simulink model "fly_gaze_sim"  (R2022a)
settings: Solver=ode45  StartTime=0.0  StopTime=t_run  MaxStep=1e-4  RelTol=1e-6
values from neighbouring files (symbols this model uses):
  frequency = test_frequencies(i)    [generate_data.m]
  t_run = 1 + 10/frequency    [generate_data.m]
libraries: simulink x1
settings Model: Creator=Ben  LastModifiedBy=Ben

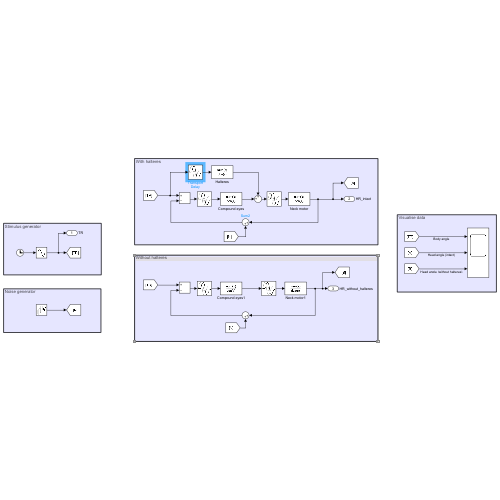
[thumbnail: Simulink's stored preview of the top-level diagram]
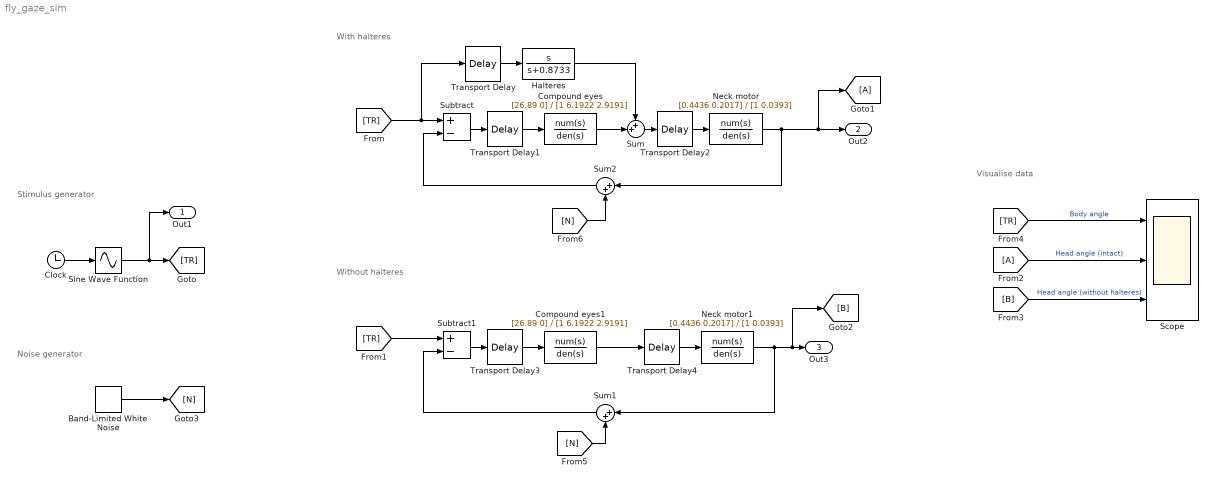
== system fly_gaze_sim ==
  note: Noise generator
  note: Visualise data
  note: With halteres
  note: Stimulus generator
  note: Without halteres
  Band-Limited White Noise : simulink/Sources/Band-Limited White Noise  Cov=[1/t_run]  Ts=0.000001*t_run  seed=[23341]
  Clock : Clock
      settings: Decimation=1000
  Compound eyes : TransferFcn  Numerator=[26.89 0]  Denominator=[1 6.1922 2.9191]
  Compound eyes1 : TransferFcn  Numerator=[26.89 0]  Denominator=[1 6.1922 2.9191]
  From2 : From
  Goto1 : Goto
  Halteres : TransferFcn  Numerator=[1 0]  Denominator=[1 0.8733]
  Neck motor : TransferFcn  Numerator=[0.4436 0.2017]  Denominator=[1 0.0393]
  Neck motor1 : TransferFcn  Numerator=[0.4436 0.2017]  Denominator=[1 0.0393]
  Scope : Scope  NumInputPorts=3
  Sine Wave Function : Sin  TimeSource=Use external signal  Amplitude=30  Frequency=frequency*pi*2  SampleTime=0
  Subtract : Sum  Inputs=+-
  Subtract1 : Sum  Inputs=+-
  Sum : Sum  Inputs=++|
  Sum1 : Sum  Inputs=|++
  Sum2 : Sum  Inputs=|++
  Transport Delay : TransportDelay  DelayTime=0.003  BufferSize=14000
  Transport Delay1 : TransportDelay  DelayTime=0.009  BufferSize=14000
  Transport Delay2 : TransportDelay  DelayTime=0.0021  BufferSize=14000
  Transport Delay3 : TransportDelay  DelayTime=0.009  BufferSize=14000
  Transport Delay4 : TransportDelay  DelayTime=0.0021  BufferSize=14000
  Out1 : Outport  SignalName=TR
  Out2 : Outport  Port=2  SignalName=HR_intact
  Out3 : Outport  Port=3  SignalName=HR_without_halteres
  wires:
  Clock/1 -> Sine Wave Function/1
  Sine Wave Function/1 -> Out1/1, [TR]
  [TR] -> Transport Delay/1, Subtract/1
  Compound eyes/1 -> Sum/2
  Halteres/1 -> Sum/1
  [TR] -> Subtract1/1
  Subtract1/1 -> Transport Delay3/1
  Neck motor1/1 -> [B], Out3/1, Sum1/1
  Compound eyes1/1 -> Transport Delay4/1
  From2/1 -> Scope/2  "Head angle (intact)"
  [B] -> Scope/3  "Head angle (without halteres)"
  [TR] -> Scope/1  "Body angle"
  Transport Delay/1 -> Halteres/1
  Transport Delay1/1 -> Compound eyes/1
  Subtract/1 -> Transport Delay1/1
  Transport Delay2/1 -> Neck motor/1
  Sum/1 -> Transport Delay2/1
  Transport Delay3/1 -> Compound eyes1/1
  Transport Delay4/1 -> Neck motor1/1
  Sum1/1 -> Subtract1/2
  Band-Limited White Noise/1 -> [N]
  [N] -> Sum1/2
  Sum2/1 -> Subtract/2
  [N] -> Sum2/2
  Neck motor/1 -> Sum2/1, Goto1/1, Out2/1
